simulink model "Task2_Question1"  (Simulink 8.1)
settings: Solver=FixedStepDiscrete  SolverMode=SingleTasking  StartTime=0.0  StopTime=inf  FixedStep=5e-05  RelTol=1e-3
undefined symbols (not defined in the file or in its folder): dfilt, gcbh, samplefreq, stemdo, upstartman
libraries: dspsigops x6, dsparch4 x4, dspsrcs4 x3, dspmathops x1
(part 1 of 2)
settings Model: Creator=hasan  LastModifiedBy=hasan
settings DataIOCC: SignalLoggingSaveFormat=Dataset  SaveOutput=off  SaveTime=off
settings OptimizationCC: BooleanDataType=off  ExpressionDepthLimit=128
settings DebuggingCC: MultiTaskDSMMsg=warning  FcnCallInpInsideContextMsg=EnableAllAsError  FrameProcessingCompatibilityMsg=none
settings GRTTargetCC: CombineOutputUpdateFcns=on  GRTInterface=off

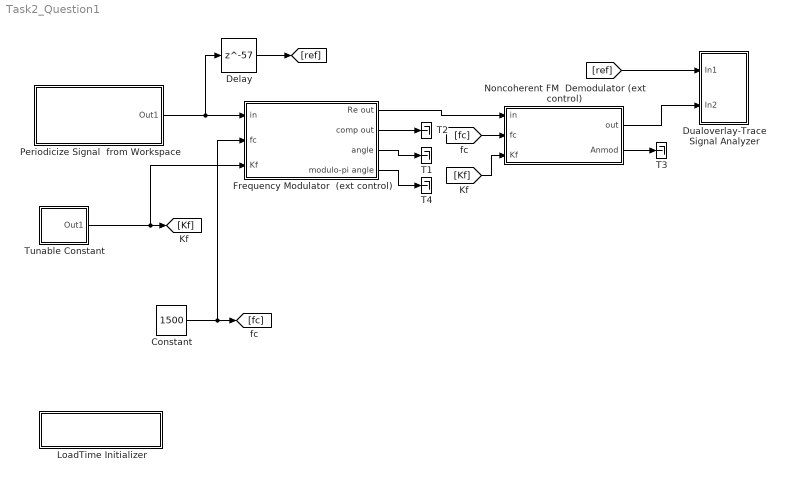
== system Task2_Question1 ==
  Constant : Constant  Value=1500
  Delay : Delay  DelayLength=57  InitialCondition=0
  Dualoverlay-Trace Signal Analyzer : Subsystem  Tag=D  Description=2-Trace Signal Analyzer (A04)  StartFcn=scopopen_April04 StartFcn  StopFcn=scopopen_April04 StopFcn  mask(2-Trace Signal Analyzer (A08)){name_plot=D, N=300, stemchoice=Continuous-plot both Inputs, V=0, nontaker=off, figpos=[0.2589 0.0583 0.6963 0.8], freqtickvec=[], strtman=off}
      mask prompts: name_plot "Name of Figure"; N "Buffer size:"; stemchoice "Plot style:"; V "Buffer overlap:"; nontaker "Override default Figure Position"; figpos "Figure Position:"; freqtickvec "Frequency-axis ticks (normally [] for default scheme)"; strtman "Startup with manual scaling"
      mask help:
      | Displays two signal vectors (depending on the choice of buffering) and their spectra. The Analyzer "name" (Name of Figure) is best assigned by clicking on the line coming into the Analyzer and labelling that line. Failing that, the dialog entry for Name of Figure is taken. If this Name collides with another Analyzer instance with the same Name, then a number is automatically added. In summary, it is permissible to give no thought to naming, unless you desire a meaningful name.
      |
      | Buffer size (typically 300) determines the number of time samples displayed and has crucial influence on stabilty of the display trace for several input sources. Both inputs (together) can either be sample-based or frame-based (when frame size matches Buffer size).
      |
      | Spectral displays can be true-zoomed in frequency (since Chirp-Z analysis is employed) via the edit boxes along the GUI bottom. By contrast, the Zoom menu item merely gives graphical zooming.
      |
      | Several controls specify the upper input port ("y" for yellow plot line) or the lower port ("w" for white plot line). Each line keeps its true vertical scaling unless temporarily overriden for VISUAL comparison purposes (see "plot scaling" menu item).
      |
      | Changes like freqtickvec and start up manual require the model to be killed and brought back up.
      | (See Help for more)
      mask init:
      | scopmsk
      settings: CopyFcn=set_param(gcb,'tag','')  DeleteFcn="scopopen_April04  DeleteFcn"  OpenFcn=scopopen_April04 OpenFcn
      mask Help:
      | Displays a signal vector (depending on the choice of buffering) and its spectrum. The Analyzer "name" (Name of Figure) is best assigned by clicking on the line coming into the Analyzer and labelling that line. Failing that, the dialog entry for Name of Figure is taken. If this Name collides with another Analyzer instance with the same Name, then a number is automatically added. In summary, it is permissible to give no thought to naming, unless you desire a meaningful name.
      | 
      | Buffer size (typically 300) determines the number of time samples displayed and has crucial influence on stabilty of the display trace for several input sources. Both inputs (together) can either be sample-based or frame-based (when frame size matches Buffer size).
      | 
      | Spectral displays can be true-zoomed in frequency (since Chirp-Z analysis is employed) via the edit boxes along the GUI bottom. By contrast, the Zoom menu item merely gives graphical zooming.
      | 
      | Several controls specify the upper input port ("y" for yellow plot line) or the lower port ("w" for white plot line). Each line keeps its true vertical scaling unless temporarily overriden for VISUAL comparison purposes (see "plot scaling" menu item).
      | 
      | Changes like freqtickvec and start up manual require the model to be killed and brought back up.
      | 
      | Dynamic amplitude scaling is automatic, but has thresholds of sensitivity (see "plot scaling" menu item) to reduce re-scale flicker . Manual re-scale (by pressing the "Full-Scale All" pushbutton is always permissible).
      | 
      | Signal (or Spectral) Averaging either uses Fading Memory from trace-to-trace (with "forgetting factor" rho unity or less) or takes each trace full-strength (over a window of N adjacent traces).
      | 
      | Copyright(c) DSP Creations Ltd. 2003-2008.
      mask TypeOptions stemchoice: Continuous-plot both Inputs | Stem-plot Input 1  [yellow]   (but 2 is continuous) | Stem-plot Input 2    [white]   (but 1 is continuous)
      mask Callback nontaker: srvscopeposition
      mask Display:
      | plot([-25 NaN 125],[0  NaN 0]);plot(0,0,100,100,[8 8 92 92 8],[92 40 40 92 92],[16 16 84],[88 48 48],[53 47 41 47 47],[34 34 34 34 21],[16 20 24 28 32 36 40 44 48 52 56 60 64 68 72 76 80],[68 74 78 80 81 80 77 73 68 64 60 58 57 57 59 63 68]);disp(name_plot);plot(0,0,100,-100,[8 8 92 92 8],-[92 40 40 92 92],[16 16 84],-[48 88 88],[24 24],-[88 58],[32 32 32],-[88 60 60],[40 40],-[88 65],[40 40],-[88 69],[48 48],-[88 80],[56 56],-[88 48],[64 64],-[88 70],[80 80 80 80],-[49 49 48 48],[53 47 47 51 47 47],-[23 23 28 28 28 34]);plot(xx,50*yy+60)
      | port_label('input',1,'y')
      | port_label('input',2,'w')
  Frequency Modulator  (ext control) : Subsystem  mask(Frequency Modulator (ext control)){thetadeg=0, sampperfr=1, twiceflag=off, conti=off, ist=off}
      mask prompts: thetadeg "Phase offset, degrees:"; sampperfr "Samples per frame"; twiceflag "Output TWICE real part (instead of Re)"; conti "Emulate continuous integration"; ist "Adopt synthetic delay-compensated time origin"
      mask help:
      | This block provides frequency modulation of a REAL signal. Both complex modulation output and real modulation are delivered.
      | The input is usually accumulated to emulate continuous-time integration. If the checkbox is on, we instead use an ABC integrator in order to more fully approximate the integration process.
      |
      | Both have had  the time origin fiddled to compensate out the group delay of the integration filter.(This is employed only if "Adopt" checkbox is ticked).
      |
      | Outputs are provided to show the instantaneous phase theta (in degrees) in exp j(2*pi*fc*t+theta(t)+ thetaoffset ), where theta emerges from our integrator  (full & modulo-pi). Note that theta seems to be on time for accumulator; must go 2 samples more for ABC integrator). That is the "comp" output.
      |
      | The real part of that is (2*pi*fc*t+theta(t)+ thetaoffset ) is delivered at the upper output port.
      | If the checkbox is ticked, then twice the real part (useful for spectral comparison) is output.
      |
      | If sample-based operation is desired then the dialog Samples per frame entry should be 1.
      |
      | The user inputs the carrier frequency through input port "fc", and the FREQUENCY SENSITIVITY (Hz/volt) through port "Kf".
      | The frequency deviation deltaf=Kf*A, when the input is a sinewave of amplitude A, as per definitions from Haykin,S.," Communication Systems",4th Edition, Wiley,2001, page 110.
      mask init:
      | sample_time_str=get_param(bdroot(gcbh),'fixedstep');
      | ts=eval(sample_time_str,'0');
      | if ts==0;
      |    samplefreq=20000;
      | else
      |    samplefreq=1/ts;
      | end;
      | a=[1 -1];
      | icvec=0;
      | b=1;
      | offs=0.5;
      | if(conti);
      |    b=[-.0099827 .0694943 .8809768  .0694943 -.0099827 ];
      |   offs=-1.5;
      | end;
      | if(~ist);offs=0;end
      | resay='Re';
      | mult=1;
      | if(twiceflag)
      | 	resay='2 Re';
      | 	mult=2;
      | end
      mask Help:
      | This block provides frequency modulation of a REAL signal. Both complex modulation output and real modulation are delivered.
      | The input is usually accumulated to emulate continuous-time integration. If the checkbox is on, we instead use an ABC integrator in order to more fully approximate the integration process.
      | 
      | Both have had  the time origin fiddled to compensate out the group delay of the integration filter.(This is employed only if "Adopt" checkbox is ticked).
      | 
      | Outputs are provided to show the instantaneous phase theta (in degrees) in exp j(2*pi*fc*t+theta(t)+ thetaoffset ), where theta emerges from our integrator  (full & modulo-pi). Note that theta seems to be on time for accumulator; must go 2 samples more for ABC integrator). That is the "comp" output.
      | 
      | The real part of that is (2*pi*fc*t+theta(t)+ thetaoffset ) is delivered at the upper output port.
      | If the checkbox is ticked, then twice the real part (useful for spectral comparison) is output.
      | 
      | If sample-based operation is desired then the dialog Samples per frame entry should be 1.
      | 
      | The user inputs the carrier frequency through input port "fc", and the FREQUENCY SENSITIVITY (Hz/volt) through port "Kf".
      | The frequency deviation deltaf=Kf*A, when the input is a sinewave of amplitude A, as per definitions from Haykin,S.," Communication Systems",4th Edition, Wiley,2001, page 110.
      | 
      | Copyright(c) DSP Creations Ltd. 2003-2013.
      mask Display:
      | disp(['Frequency\nModulator\nthetaoffset = ',num2str(thetadeg)])
      | port_label('input',1,'in')
      | port_label('input',2,'fc')
      | port_label('input',3,'Kf')
      | port_label('output',1,resay)
      | port_label('output',2,'comp')
      | port_label('output',3,'angle')
      | port_label('output',4,'mod-pi ang')
  LoadTime Initializer : Subsystem  Description="Click on block OR right-click and select \"Mask Parameters...\" for description of block."  InitFcn=eval(['load ',get_param(gcbh,'filename')])  mask(LoadTime Initializer){filename=bussgangwanderwave}
      mask prompts: filename "Specify MAT filename to load"
      mask help: Insertion of this block into a model ensures loading of the specified mat-file at load time.
      mask init:
      | linkbreakergraceful
      | eval(['load ',filename])
      mask Help:
      | Insertion of this block into a model ensures loading of the specified mat-file at load time.
      | 
      | 14_feb11
      | Copyright(c) DSP Creations Ltd. 2003-2014.
      mask Callback filename: eval(['load ',get_param(gcbh,'filename')])
      mask Display: disp(['Initialize\n '' ',filename,' '''])
  Noncoherent FM  Demodulator (ext control) : Subsystem  mask(Noncoherent FM Demodulator (ext control)){dclength=300, incomplex=off, iee=off}
      mask prompts: dclength "D.c. bias removal data block length"; incomplex "Take input as fully complex"; iee "Compensate emulation of continuous integration"
      mask help:
      | This block provides non-coherent demodulation of a real cosine frequency-modulated carrier OR frequency-modulated complex sinusoidal carrier.
      | If a fully complex input situation is known to prevail, then check  "Take input as fully complex " (which disturbs the input minimally).
      |
      | The Analyticized modulation signal is provided for viewing at the "Anmod" output port.
      |     (In case  "Take input as fully complex" is ticked, the unmodified input signal will be seen as "Anmod" ).
      |
      | The user inputs the carrier frequency through input port "fc", and the FREQUENCY SENSITIVITY (Hz/volt) through port "Kf".
      | The frequency deviation deltaf=Kf*A, when the input is a sinewave of amplitude A, as per definitions from Haykin,S.," Communication Systems",4th Edition, Wiley,2001, page 110.
      |
      | If for any reason you wish to remove all d.c. from any output, place an integer number in for "D.c. bias removal data block length". If you are satisfied with the d.c. value, instead place empty brackets for this value.
      |
      | NOTE: There is an internal 100-sample delay due to the necessary high-grade Analytic filtering. HOWEVER, if input is taken as complex there is zero delay.
      |
      | Usually the original FM signal was created by accumulation, so output is okay. But you might be working with FM where "continuous integration" had been emulated; if so, tick the last checkbox (dubious improvement).
      |
      | This demodulator requires no major bandwidth assumptions. However, the Analytic filter will give distortion if the lower bandedge of the bandpass modulation signal input is below 0.037*fs or above 0.466*fs.
      mask init:
      | linkbreakergraceful;
      | sample_time_str=get_param(bdroot(gcbh),'fixedstep');
      | ts=eval(sample_time_str,'0');
      | if ts==0;
      |    samplefreq=20000;
      | else
      |    samplefreq=1/ts;
      | end;
      | saystr=['Noncoherent FM\nDemodulator'];
      | lengthflag=0;
      | block=1;
      | if(~isempty(dclength))
      |    lengthflag=1;
      |    block=dclength;
      |    saystr=[saystr '\nd.c. remove ',num2str(dclength),'\n'];
      | end
      | bcomp=1;
      | if(iee);
      |    bint=[-.0099827 .0694943 .8809768  .0694943 -.0099827 ];
      |    bcomp=firinvleastsq(bint);
      | end;
      | insay='in';
      | if(incomplex)
      |    insay='comp in';
      | end
      mask Help:
      | This block provides non-coherent demodulation of a real cosine frequency-modulated carrier OR frequency-modulated complex sinusoidal carrier.
      | If a fully complex input situation is known to prevail, then check  "Take input as fully complex " (which disturbs the input minimally).
      | 
      | The Analyticized modulation signal is provided for viewing at the "Anmod" output port.
      |     (In case  "Take input as fully complex" is ticked, the unmodified input signal will be seen as "Anmod" ).
      | 
      | The user inputs the carrier frequency through input port "fc", and the FREQUENCY SENSITIVITY (Hz/volt) through port "Kf".
      | The frequency deviation deltaf=Kf*A, when the input is a sinewave of amplitude A, as per definitions from Haykin,S.," Communication Systems",4th Edition, Wiley,2001, page 110.
      | 
      | If for any reason you wish to remove all d.c. from any output, place an integer number in for "D.c. bias removal data block length". If you are satisfied with the d.c. value, instead place empty brackets for this value.
      | 
      | NOTE: There is an internal 100-sample delay due to the necessary high-grade Analytic filtering. HOWEVER, if input is taken as complex there is zero delay.
      | 
      | Usually the original FM signal was created by accumulation, so output is okay. But you might be working with FM where "continuous integration" had been emulated; if so, tick the last checkbox (dubious improvement).
      | 
      | This demodulator requires no major bandwidth assumptions. However, the Analytic filter will give distortion if the lower bandedge of the bandpass modulation signal input is below 0.037*fs or above 0.466*fs.
      | 
      | 14_May5
      | Copyright(c) DSP Creations Ltd. 2003-2014.
      mask Display:
      | disp(saystr)
      | port_label('input',1,insay)
      | port_label('input',2,'fc')
      | port_label('input',3,'Kf')
      | port_label('output',1,'out')
      | port_label('output',2,'Anmod')
  Periodicize Signal  from Workspace : Subsystem  mask(Arbitrary Periodic Signal Generator){signal_name_str=bussgangwanderwave, A=1, Ntry=[], dwellsamp=1, fill0=off}
      mask prompts: signal_name_str "Signal name (in workspace)"; A "Amplification, A"; Ntry "Period, N (=[ ] if same as length of signal)"; dwellsamp "Dwell interval (in samples) before stepping to next sample of signal"; fill0 "Fill interval between signal samples with zeros (instead of holding)"
      mask help:
      | This takes a vector signal in the workspace as the base period for a periodic signal. Note that a short period can time-alias the base period. At present, no special icon indication comes if the signal is complex.
      |
      | This signal generator is analogous to a Refresh DAC; it loads in (from the Workspace or from its dialog box) a (real or complex) signal vector and then repeatedly clocks it out. We have really a causal periodic buildup. Normally you let the vector "Signal name" dictate the period (to be length of signal_name) by leaving "Period" empty, but this can be set longer or (if shorter) to time-alias. Note that a vector of numbers can be used in place of a vector name in the dialog box.
      |
      | Dwell interval (usually 1 when stepping right through signal samples), dwellsamp, can be set to an integer value. This then holds the signal value constant for dwellsamp clock times before moving on to take the next sample explicitly set out in  the vector signal name.
      | Thus, the true period taken to cycle through the signal is  Period*dwellsamp.
      |
      | If the checkbox is ticked the dwellsample interval between specified signal samples is filled with zeros; otherwise values are held for whole interval.
      mask init:
      | maskmaster('passkey_integerize','Ntry',Ntry);
      | sample_time_str=get_param(bdroot(gcbh),'fixedstep');
      | ts=eval(sample_time_str,'0');
      | if ts==0;
      |    samplefreq=20000;
      | else
      |    samplefreq=1/ts;
      | end;
      | signal_name=evalin('base',signal_name_str,'[1:4]');
      | Ns=length(signal_name);
      | if(isempty(Ntry))
      |    N=Ns;
      | else
      |    N=Ntry;
      | end
      | if(Ns<=N);
      |     x=[signal_name  zeros(1,N-Ns)];
      | else;
      |     innn=[signal_name zeros(1,Ns+2*N)];
      |     opt=filter(1,[1 zeros(1,N-1) -1],innn);
      |     x=opt(length(signal_name)+1:Ns+2*N);
      | end
      | iflag=0;
      | if(any(imag(x)))
      |   iflag=1;
      | end
      | if(isreal(x))
      |   d2=['total cycle= ' num2str(N*dwellsamp)];
      | else	
      |   d2=['total cycle= ' num2str(N*dwellsamp),'   (Re seen)'];
      | end
      | dwellsamp=floor(abs(dwellsamp));
      | gg=real(x);
      | Lg=length(gg);
      | rr=repmat(gg,dwellsamp,1);
      | zerodo=0;
      | if(strcmp(fill0,'on'));
      | 	zerodo=1;	
      |    rr=[gg; zeros(dwellsamp-1,Lg)];
      | end 
      | gg=reshape(rr,1,dwellsamp*Lg);
      | if(length(gg)>2000)
      |    dec=ceil(length(gg)/2000);
      |    gg=gg(1:dec:end);
      | end	
      | mm=max(gg);
      | mi=min(gg);
      | Ngg=length(gg);
      mask Help:
      | This takes a vector signal in the workspace as the base period for a periodic signal. Note that a short period can time-alias the base period. At present, no special icon indication comes if the signal is complex.
      | 
      | This signal generator is analogous to a Refresh DAC; it loads in (from the Workspace or from its dialog box) a (real or complex) signal vector and then repeatedly clocks it out. We have really a causal periodic buildup. Normally you let the vector "Signal name" dictate the period (to be length of signal_name) by leaving "Period" empty, but this can be set longer or (if shorter) to time-alias. Note that a vector of numbers can be used in place of a vector name in the dialog box.
      | 
      | Dwell interval (usually 1 when stepping right through signal samples), dwellsamp, can be set to an integer value. This then holds the signal value constant for dwellsamp clock times before moving on to take the next sample explicitly set out in  the vector signal name.
      | Thus, the true period taken to cycle through the signal is  Period*dwellsamp.
      | 
      | If the checkbox is ticked the dwellsample interval between specified signal samples is filled with zeros; otherwise values are held for whole interval.
      | 
      | 14_Feb12
      | Copyright(c) DSP Creations Ltd. 2003-2014.
      mask Display:
      | plot(.02+.96*[0:Ngg-1]/(Ngg-1),.28+.6*(gg-mi)/(mm-mi))
      | text(.02,.9,[signal_name_str,' periodicized'])
      | text(.02,.255,['period= ' num2str(N) ' samples'])
      | text(.02,.085,d2)
  T{1..4} (4 alike) : Terminator
  Tunable Constant : Subsystem  LoadFcn=slideg Load  mask(Tunable Constant){low=0, gain=3397, high=3397}
      mask help: This signal generator gives out a constant value which is slider-adjustable.
      mask init:
      | %set_param(gcb,'linkstatus','none');
      | if(~strcmp(get_param(gcb,'linkstatus'),'none'))
      |    set_param(gcb,'linkstatus','none');	
      | end
      | sample_freq=maskmaster('Sinusoid Generator',1);
      settings: CopyFcn=slideg Copy  DeleteFcn=slideg DeleteBlock  NameChangeFcn=slideg NameChange  OpenFcn=slideg Open  CloseFcn=slideg Close  ParentCloseFcn=slideg ParentClose
      mask Help:
      | This signal generator gives out a constant value which is slider-adjustable.
      | 
      | Copyright(c) DSP Creations Ltd. 2003-2013.
      mask Display: disp(gain)
  wires:
  Frequency Modulator  (ext control)/2(comp out) -> T2/1
  Frequency Modulator  (ext control)/3(angle) -> T1/1
  Frequency Modulator  (ext control)/4(modulo-pi angle) -> T4/1
  Noncoherent FM  Demodulator (ext control)/2(Anmod) -> T3/1
  Periodicize Signal  from Workspace/1(Out1) -> Delay/1, Frequency Modulator  (ext control)/1(in)
  Frequency Modulator  (ext control)/1(Re out) -> Noncoherent FM  Demodulator (ext control)/1(in)
  Constant/1 -> [fc], Frequency Modulator  (ext control)/2(fc)
  Delay/1 -> [ref]
  [ref] -> Dualoverlay-Trace Signal Analyzer/1(In1)
  Noncoherent FM  Demodulator (ext control)/1(out) -> Dualoverlay-Trace Signal Analyzer/2(In2)
  Tunable Constant/1(Out1) -> [Kf], Frequency Modulator  (ext control)/3(Kf)
  [fc] -> Noncoherent FM  Demodulator (ext control)/2(fc)
  [Kf] -> Noncoherent FM  Demodulator (ext control)/3(Kf)

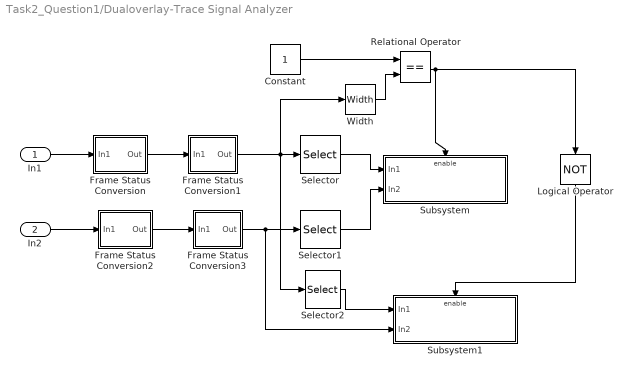
== system Task2_Question1/Dualoverlay-Trace Signal Analyzer ==
  In1 : Inport
  In2 : Inport  Port=2
  Constant : Constant
  Frame Status Conversion : Subsystem  mask(Frame Status Conversion){growRefPort=off, outframe=Frame-based}
      mask prompts: growRefPort "Inherit output frame status from Ref input port"; outframe "Output signal:"
      mask help: Specify the frame status of the output signal.
      mask init:
      | [p, str] = dspblkfrmconv('init');
      mask Help: web(dspbhelp);
      mask Callback growRefPort: dspblkfrmconv
      mask TypeOptions outframe: Frame-based | Sample-based
      mask Display:
      | port_label(p.in1,   p.i1,  p.i1s);
      | port_label(p.in2,   p.i2,  p.i2s);
      | port_label(p.out, p.o1, p.o1s);
      | disp(str)
  Frame Status Conversion1 : Subsystem  mask(Frame Status Conversion){growRefPort=off, outframe=Sample-based}
      mask prompts: growRefPort "Inherit output frame status from Ref input port"; outframe "Output signal:"
      mask help: Specify the frame status of the output signal.
      mask init:
      | [p, str] = dspblkfrmconv('init');
      mask Help: web(dspbhelp);
      mask Callback growRefPort: dspblkfrmconv
      mask TypeOptions outframe: Frame-based | Sample-based
      mask Display:
      | port_label(p.in1,   p.i1,  p.i1s);
      | port_label(p.in2,   p.i2,  p.i2s);
      | port_label(p.out, p.o1, p.o1s);
      | disp(str)
  Frame Status Conversion2 : Subsystem  mask(Frame Status Conversion){growRefPort=off, outframe=Frame-based}
      mask prompts: growRefPort "Inherit output frame status from Ref input port"; outframe "Output signal:"
      mask help: Specify the frame status of the output signal.
      mask init:
      | [p, str] = dspblkfrmconv('init');
      mask Help: web(dspbhelp);
      mask Callback growRefPort: dspblkfrmconv
      mask TypeOptions outframe: Frame-based | Sample-based
      mask Display:
      | port_label(p.in1,   p.i1,  p.i1s);
      | port_label(p.in2,   p.i2,  p.i2s);
      | port_label(p.out, p.o1, p.o1s);
      | disp(str)
  Frame Status Conversion3 : Subsystem  mask(Frame Status Conversion){growRefPort=off, outframe=Sample-based}
      mask prompts: growRefPort "Inherit output frame status from Ref input port"; outframe "Output signal:"
      mask help: Specify the frame status of the output signal.
      mask init:
      | [p, str] = dspblkfrmconv('init');
      mask Help: web(dspbhelp);
      mask Callback growRefPort: dspblkfrmconv
      mask TypeOptions outframe: Frame-based | Sample-based
      mask Display:
      | port_label(p.in1,   p.i1,  p.i1s);
      | port_label(p.in2,   p.i2,  p.i2s);
      | port_label(p.out, p.o1, p.o1s);
      | disp(str)
  Logical Operator : Logic  Operator=NOT
  Relational Operator : RelationalOperator  Operator===  InputSameDT=on
  Selector : Selector  NumberOfDimensions=2  InputPortWidth=3  IndexOptions=Index vector (dialog),Index vector (dialog)  Indices=1,1  OutputSizes=1
  Selector1 : Selector  NumberOfDimensions=2  InputPortWidth=3  IndexOptions=Index vector (dialog),Index vector (dialog)  Indices=1,1  OutputSizes=1
  Selector2 : Selector  NumberOfDimensions=2  InputPortWidth=3  IndexOptions=Select all,Index vector (dialog)  Indices=-1,1  OutputSizes=1
  Subsystem : Subsystem  TreatAsAtomicUnit=on
  Subsystem1 : Subsystem  TreatAsAtomicUnit=on
  Width : Width
  wires:
  Selector1/1 -> Subsystem/2(In2)
  Selector/1 -> Subsystem/1(In1)
  Selector2/1 -> Subsystem1/1(In1)
  Logical Operator/1 -> Subsystem1/Enable
  Relational Operator/1 -> Logical Operator/1, Subsystem/Enable
  Width/1 -> Relational Operator/2
  Constant/1 -> Relational Operator/1
  Frame Status Conversion3/1(Out) -> Subsystem1/2(In2), Selector1/1
  In2/1 -> Frame Status Conversion2/1(In1)
  Frame Status Conversion2/1(Out) -> Frame Status Conversion3/1(In1)
  Frame Status Conversion1/1(Out) -> Selector2/1, Selector/1, Width/1
  In1/1 -> Frame Status Conversion/1(In1)
  Frame Status Conversion/1(Out) -> Frame Status Conversion1/1(In1)

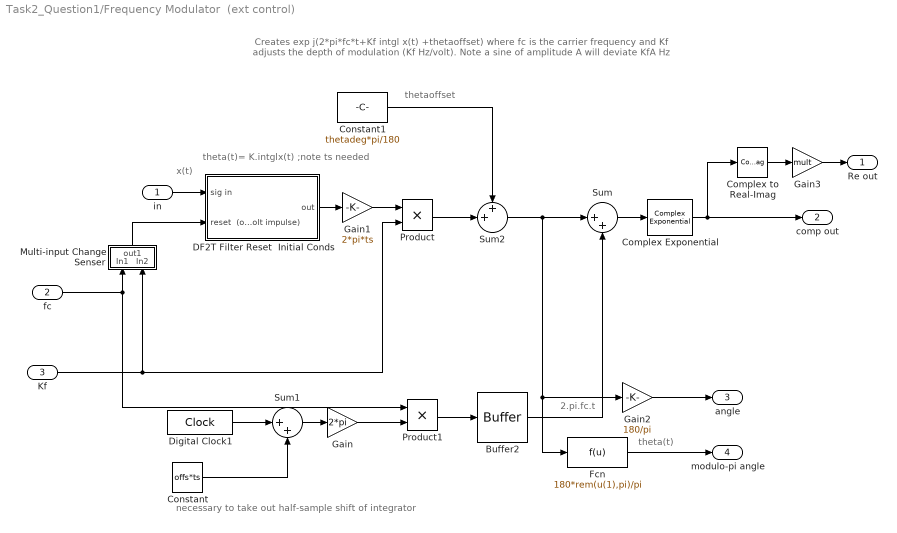
== system Task2_Question1/Frequency Modulator  (ext control) ==
  note: thetaoffset
  note: x(t)
  note: Creates exp j(2*pi*fc*t+Kf intgl x(t) +thetaoffset) where fc is  the carrier frequency
      |  and Kf adjusts the depth of modulation (Kf Hz/volt).
      |  Note a sine of amplitude A will deviate KfA Hz
  note: 2.pi.fc.t
  note: theta(t)=
      | K.intglx(t) ;note ts needed
  note: necessary to take out
      |  half-sample shift of integrator
  note: theta(t)
  in : Inport
  fc : Inport  Port=2
  Kf : Inport  Port=3
  Buffer2 : Buffer  N=sampperfr
  Complex Exponential : dspmathops/Complex Exponential
  Complex to Real-Imag : ComplexToRealImag  Output=Real
  Constant : Constant  Value=offs*ts
  Constant1 : Constant  Value=thetadeg*pi/180
  DF2T Filter Reset  Initial Conds : Subsystem  mask(Direct Form 2 Transpose Filter Reset Initial Conds){b=b, a=a, Xicvec=0, Yicvec=0}
      mask prompts: b "Numerator coefficient vector, b"; a "Denominator coefficient vector, a"; Xicvec "Vector of  INPUT x initial conditions, Xicvec:"; Yicvec "Vector of  OUTPUT y initial conditions, Yicvec:"
      mask help:
      | This block has resettable initial conditions, making it possible to exhibit stationary repetitive displays of the effects of ic's, perhaps even as coefficients are tuned.
      |
      | The b and a filter  coefficients are input as vector parameters.
      | The initial condition vectors  are fed in in this form:
      |    Xicvec = [ x[-1] x[-2] x[-3] ... x[-nb] ... ]   (inputs)
      |    Yicvec = [ y[-1] y[-2] y[-3] ... y[-na] ... ]    (outputs)
      |
      | (These are packaged for DF2T as a chain of delayor ic's internal to the block, using MATLAB's filtic command).
      |
      | The output of the filter is delayed by one bulk sample  since, internal to this block, the reset has to initiate immediately (before data flow).
      | (That is, the first sample out of the filter is actually y(-1), so there is a pervasive delay of the time scale by one sample.
      |
      | Resetting is achieved by a unit-amplitude impulse.
      mask init:
      | icvec=filtic(b,a,Yicvec,Xicvec);
      | sample_time_str=get_param(bdroot(gcbh),'fixedstep');
      | ts=eval(sample_time_str,'0');
      | if ts==0;
      |    samplefreq=20000;
      | else
      |    samplefreq=1/ts;
      | end;
      mask Help:
      | This block has resettable initial conditions, making it possible to exhibit stationary repetitive displays of the effects of ic's, perhaps even as coefficients are tuned.
      | 
      | The b and a filter  coefficients are input as vector parameters.
      | The initial condition vectors  are fed in in this form:
      |    Xicvec = [ x[-1] x[-2] x[-3] ... x[-nb] ... ]   (inputs)
      |    Yicvec = [ y[-1] y[-2] y[-3] ... y[-na] ... ]    (outputs)
      | 
      | (These are packaged for DF2T as a chain of delayor ic's internal to the block, using MATLAB's filtic command).
      | 
      | The output of the filter is delayed by one bulk sample  since, internal to this block, the reset has to initiate immediately (before data flow).
      | (That is, the first sample out of the filter is actually y(-1), so there is a pervasive delay of the time scale by one sample.
      | 
      | Resetting is achieved by a unit-amplitude impulse.
      | 
      | Copyright(c) DSP Creations Ltd. 2003-2006.
      mask Display:
      | disp('Direct Form 2T\nReset Initial\nCond Filter')
      | port_label('input',1,'in')
      | port_label('input',2,'reset')
  Digital Clock1 : DigitalClock  SampleTime=ts
  Fcn : Fcn  Expr=180*rem(u(1),pi)/pi
  Gain : Gain  Gain=2*pi  SaturateOnIntegerOverflow=on  OutDataTypeStr=Inherit: Same as input  ParamDataTypeStr=Inherit: Same as input
  Gain1 : Gain  Gain=2*pi*ts  SaturateOnIntegerOverflow=on  OutDataTypeStr=Inherit: Same as input  ParamDataTypeStr=Inherit: Same as input
  Gain2 : Gain  Gain=180/pi  SaturateOnIntegerOverflow=on  OutDataTypeStr=Inherit: Same as input  ParamDataTypeStr=Inherit: Same as input
  Gain3 : Gain  Gain=mult  SaturateOnIntegerOverflow=on  OutDataTypeStr=Inherit: Same as input  ParamDataTypeStr=Inherit: Same as input
  Multi-input Change Senser : Subsystem  Description=Multi-Input Change Senser  mask(Multi-input Change Senser){vector=[1 2]}
      mask prompts: vector "Channel Values Vector"
      mask help:
      | This block detects any change on any of its input ports (including at startup) and issues a unit-voltage impulse.
      |
      | The syntax for the Channel Values Vector is, e.g.: [1 2 3 4] or [5 8]:
      |
      | WARNING: Any block housing this block should itself initialize with set_param(gcb,'linkstatus','none');
      mask init:
      | set_param(gcb,'linkstatus','none');
      mask Help:
      | This block detects any change on any of its input ports (including at startup) and issues a unit-voltage impulse.
      | 
      | The syntax for the Channel Values Vector is, e.g.: [1 2 3 4] or [5 8]:
      | 
      | WARNING: Any block housing this block should itself initialize with set_param(gcb,'linkstatus','none');
      | 
      | Copyright(c) DSP Creations Ltd. 2003-2010.
      mask Callback vector: udscope3d_forsenser
      mask Display: port_label('input',1,'1'),port_label('input',2,'2'),
  Product : Product  SaturateOnIntegerOverflow=on  OutDataTypeStr=Inherit: Same as first input
  Product1 : Product  SaturateOnIntegerOverflow=on  OutDataTypeStr=Inherit: Same as first input
  Sum : Sum  Inputs=|++  SaturateOnIntegerOverflow=on  InputSameDT=on  OutDataTypeStr=Inherit: Same as first input
  Sum1 : Sum  Inputs=|++  SaturateOnIntegerOverflow=on  InputSameDT=on  OutDataTypeStr=Inherit: Same as first input
  Sum2 : Sum  Inputs=++|  SaturateOnIntegerOverflow=on  InputSameDT=on  OutDataTypeStr=Inherit: Same as first input
  Re out : Outport  InitialOutput=0
  comp out : Outport  Port=2  InitialOutput=0
  angle : Outport  Port=3  InitialOutput=0
  modulo-pi angle : Outport  Port=4  InitialOutput=0
  wires:
  fc/1 -> Product1/1, Multi-input Change Senser/1(In1)
  Product1/1 -> Buffer2/1
  Gain/1 -> Product1/2
  Kf/1 -> Multi-input Change Senser/2(In2), Product/2
  Product/1 -> Sum2/2
  Gain1/1 -> Product/1
  Multi-input Change Senser/1(out1) -> DF2T Filter Reset  Initial Conds/2(reset  (one-volt impulse))
  Constant1/1 -> Sum2/1
  Sum2/1 -> Gain2/1, Fcn/1, Sum/1
  Gain3/1 -> Re out/1
  Complex to Real-Imag/1 -> Gain3/1
  Complex Exponential/1 -> Complex to Real-Imag/1, comp out/1
  in/1 -> DF2T Filter Reset  Initial Conds/1(sig in)
  DF2T Filter Reset  Initial Conds/1(out) -> Gain1/1
  Sum/1 -> Complex Exponential/1
  Fcn/1 -> modulo-pi angle/1
  Gain2/1 -> angle/1
  Digital Clock1/1 -> Sum1/1
  Sum1/1 -> Gain/1
  Constant/1 -> Sum1/2
  Buffer2/1 -> Sum/2

== system Task2_Question1/LoadTime Initializer ==

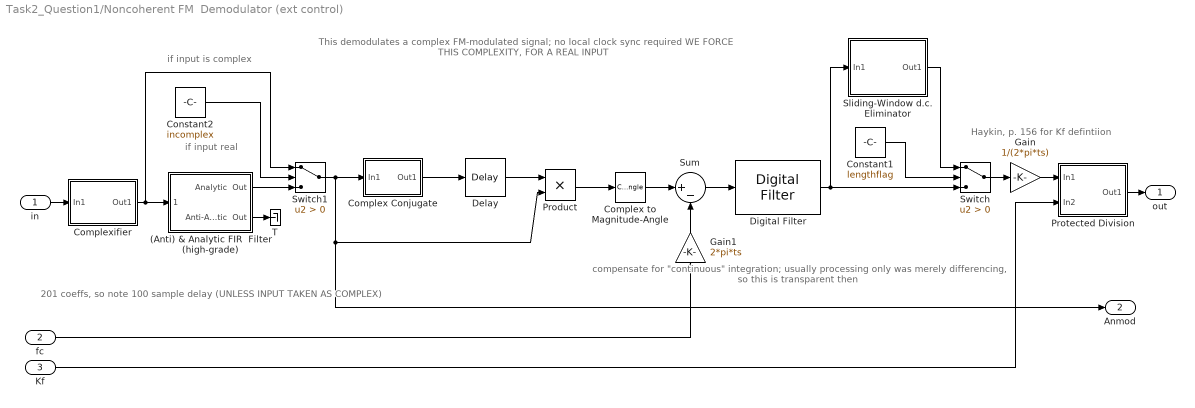
== system Task2_Question1/Noncoherent FM  Demodulator (ext control) ==
  note: This demodulates a complex FM-modulated signal; no local clock sync required
      | WE FORCE THIS COMPLEXITY, FOR A REAL INPUT
  note: compensate for "continuous" integration;
      | usually processing only was
      |  merely differencing, so this is
      | transparent then
  note: Haykin, p. 156
      |  for Kf defintiion
  note: 201 coeffs, so note
      |  100 sample delay
      | (UNLESS INPUT
      |  TAKEN AS COMPLEX)
  note: if input is complex
  note: if input real
  in : Inport
  fc : Inport  Port=2
  Kf : Inport  Port=3
  (Anti) & Analytic FIR  Filter (high-grade) : Subsystem  Description=|  mask((Anti) and Analytic FIR Filter (high-grade)){icvec=0, opcoeffs=off}
      | This block filters just like MATLAB's filter command.The b coefficient vector is either typed in-place numerically or is the name of some vector in the Workspace.
      |                                                                                                                                                                   
      | Initial conditions are always zero.                                                                                                                               
      |                                                                                                                                                                   
      | A checkbox allows normalization of the impulse response to unit energy. A second checkbox allows creation of a port for output of the b coefficient vector.       
      |                                                                                                                                                                   
      | Copyright(c) DSP Creations Ltd. 2003-2004.
      mask prompts: icvec "Vector of  INPUT x initial conditions, Xicvec:"; opcoeffs "Output Filter Coefficients"
      mask help:
      | This block provides high-grade Analytic filtering from the upper output port. That is, for negative frequencies the gain is zero, while it is 2 for positive frequencies.
      | This a fixed design, with 201 coefficients; it has linear phase and a delay of 100 samples.
      |
      | Error is less than 0.000003 from frequency of 0.037*fs to 0.466*fs , and about symmetrically.
      | Thus, if you can live with the bandlimitedness, the quality is excellent.
      |
      | The initial condition vectors  are fed in in this form:
      |    Xicvec = [ x[-1] x[-2] x[-3] ... x[-nb] ... ]   (inputs)
      |
      | A checkbox allows creation of a port for output of the b coefficient vector.
      mask init:
      | b=analyticFIRhighgrade;
      | gg=gain(b,1);
      | if(length(gg)>2000)
      |    dec=ceil(length(gg)/2000);
      |    gg=gg(1:dec:end);
      | end	
      | mm=max(gg);
      mask Help:
      | This block provides high-grade Analytic filtering. That is, for negative frequencies the gain is zero, while it is 2 for positive frequencies.
      | This a fixed design, with 201 coefficients; it has linear phase and a delay of 100 samples.
      | 
      | Error is less than 0.000003 from frequency of 0.037*fs to 0.466*fs , and about symmetrically.
      | Thus, if you can live with the bandlimitedness, the quality is excellent.
      | 
      | The initial condition vectors  are fed in in this form:
      |    Xicvec = [ x[-1] x[-2] x[-3] ... x[-nb] ... ]   (inputs)
      | 
      | A checkbox allows creation of a port for output of the b coefficient vector.
      | 
      | Copyright(c) DSP Creations Ltd. 2003-2007.
      mask Callback opcoeffs: constructoutputs(gcb,1)
      mask Display:
      | color('blue');
      | plot([1.1*mm nan gg nan -0.1])
      | color('black');
      | text(0,-.2*mm,[' Analytic, N=201'])
      | text(0,-.4*mm,[' '])
  Complex Conjugate : Subsystem  mask(Complex Conjugate){}
      mask help: This block forms the complex conjugate of its input.
      mask Help:
      | This block forms the complex conjugate of its input.
      | 
      | Copyright(c) DSP Creations Ltd. 2003-2004.
      mask Display: disp('*\nConjugate' )
  Complex to Magnitude-Angle : ComplexToMagnitudeAngle  Output=Angle
  Complexifier : Subsystem  mask(Phoney Complexifier){}
      mask help: This utility block makes its input complex even if real. It is sometimes useful for interfacing simultaneous input with mixed real and complex types.
      mask Help:
      | This utility block makes its input  complex even if real. It is sometimes useful for interfacing simultaneous input with mixed real and complex types.
      | 
      | Copyright(c) DSP Creations Ltd. 2003-2004.
      mask Display: disp('Phoney\nComplexifier')
  Constant1 : Constant  Value=lengthflag
  Constant2 : Constant  Value=incomplex
  Delay : dspsigops/Delay  InputProcessing=Inherited (this choice will be removed - see release notes)  dly_unit=Samples  delay=1  ic_detail=off  dif_ic_for_ch=off  dif_ic_for_dly=off  ic=0  reset_popup=None
  Digital Filter : dsparch4/Digital Filter  TypePopup=FIR (all zeros)  IIRFiltStruct=Direct form II transposed  AllPoleFiltStruct=Direct form  FIRFiltStruct=Direct form  CoeffSource=Specify via dialog  NumCoeffs=bcomp  DenCoeffs=bcomp  BiQuadCoeffs=[1 0.3 0.4 1 0.1 0.2]  LatticeCoeffs=[0.2 0.4]  denIgnore=on  FiltPerSampPopup=One filter per frame  IC=0  ICnum=0  ICden=0  roundingMode=Floor  overflowMode=off  ScaleValues=1  scaleValueFracLength=14  stageInFracLength=15  stageOutFracLength=15  FilterSource=Specify via dialog  dfiltObjectName=dfilt.dffir([1 2 1])  InputProcessing=Inherited (this choice will be removed - see release notes)
  Gain : Gain  Gain=1/(2*pi*ts)  SaturateOnIntegerOverflow=on  OutDataTypeStr=Inherit: Same as input  ParamDataTypeStr=Inherit: Same as input
  Gain1 : Gain  Gain=2*pi*ts  SaturateOnIntegerOverflow=on  OutDataTypeStr=Inherit: Same as input  ParamDataTypeStr=Inherit: Same as input
  Product : Product  SaturateOnIntegerOverflow=on  InputSameDT=on  OutDataTypeStr=Inherit: Same as first input
  Protected Division : Subsystem  mask(Safe Divider){}
      mask help: This utility block protects against division by zero. The output holds at its last value whenever input "denom" takes on value zero. On the initial clock instant the output is made zero. Otherwise the output is num/denom.
      mask init:
      | linkbreakergraceful;
      mask Help:
      | This utility block protects against division by zero. The output holds at its last value whenever input "denom" takes on value zero. On the initial clock instant the output is made zero. Otherwise the output is num/denom.
      | 
      | 14_March5
      | Copyright(c) DSP Creations Ltd. 2003-2014.
      mask Display:
      | disp('\nSafe Divider\n')
      | port_label('input',1,'num')
      | port_label('input',2,'denom')
  Sliding-Window d.c. Eliminator : Subsystem  mask(Sliding Block D.C. Eliminator){N=block}
      mask prompts: N "Data block length, N"
      mask help:
      | This block removes the d.c. content from a block of data N units long. The removal is done sample-by-sample, on a sliding-window basis (with N the window length).
      |
      | The output is the current sample minus the average of all N values preceeding (and including) this sample.
      mask init:
      | sample_time_str=get_param(bdroot(gcbh),'fixedstep');
      | ts=eval(sample_time_str,'0');
      | if ts==0;
      |    samplefreq=20000;
      | else
      |    samplefreq=1/ts;
      | end;
      mask Help:
      | This block removes the d.c. content from a block of data N units long. The removal is done sample-by-sample, on a sliding-window basis (with N the window length).
      | 
      | The output is the current sample minus the average of all N values preceeding (and including) this sample.
      | 
      | Copyright(c) DSP Creations Ltd. 2003-2012.
      mask Display: disp(['N= ',num2str(N),' size\nBlock d.c.\nEliminator'])
  Sum : Sum  Inputs=|+-  SaturateOnIntegerOverflow=on  InputSameDT=on  OutDataTypeStr=Inherit: Same as first input
  Switch : Switch  Criteria=u2 > Threshold  SaturateOnIntegerOverflow=on
  Switch1 : Switch  Criteria=u2 > Threshold  SaturateOnIntegerOverflow=on
  T : Terminator
  out : Outport
  Anmod : Outport  Port=2
  wires:
  fc/1 -> Gain1/1
  Gain1/1 -> Sum/2
  Complex to Magnitude-Angle/1 -> Sum/1
  Kf/1 -> Protected Division/2(In2)
  Gain/1 -> Protected Division/1(In1)
  Protected Division/1(Out1) -> out/1
  Complexifier/1(Out1) -> Switch1/1, (Anti) & Analytic FIR  Filter (high-grade)/1(" ")
  Sliding-Window d.c. Eliminator/1(Out1) -> Switch/1
  Constant1/1 -> Switch/2
  Switch/1 -> Gain/1
  Product/1 -> Complex to Magnitude-Angle/1
  Sum/1 -> Digital Filter/1
  Digital Filter/1 -> Sliding-Window d.c. Eliminator/1(In1), Switch/3
  Delay/1 -> Product/1
  Complex Conjugate/1(Out1) -> Delay/1
  in/1 -> Complexifier/1(In1)
  Switch1/1 -> Anmod/1, Product/2, Complex Conjugate/1(In1)
  (Anti) & Analytic FIR  Filter (high-grade)/1(Analytic  Out) -> Switch1/3
  Constant2/1 -> Switch1/2
  (Anti) & Analytic FIR  Filter (high-grade)/2(Anti-Analytic  Out) -> T/1

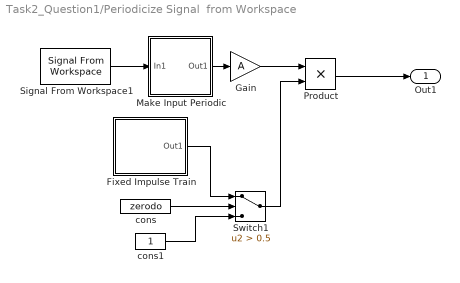
== system Task2_Question1/Periodicize Signal  from Workspace ==
  Fixed Impulse Train : Subsystem  mask(Fixed Impulse Train){N=dwellsamp}
      mask prompts: N "Repetition Period, N:"
      mask help:
      | A periodic train of unit-amplitude impulses is provided.
      |
      | This signal generator gives a unit-amplitude impulse every N samples. Intervening samples are zero-valued.
      mask init:
      | if(isempty(N))
      |     errordlg('ERROR: this value must be set to a positive integer',gcb,'modal')
      | else
      |    maskmaster('passkey_integerize','N',N)
      | end
      | sample_time_str=get_param(bdroot(gcbh),'fixedstep');
      | ts=eval(sample_time_str,'0');
      | if ts==0;
      |    samplefreq=20000;
      | else
      |    samplefreq=1/ts;
      | end;
      mask Help:
      | A periodic train of unit-amplitude impulses is provided.
      | 
      | This signal generator gives a unit-amplitude impulse every N samples. Intervening samples are zero-valued.
      | 
      | Copyright(c) DSP Creations Ltd. 2003-2004
      mask Display: disp(['Fixed Impulse\nTrain,\n Period:\n N= ',num2str(N)])
  Gain : Gain  Gain=A  SaturateOnIntegerOverflow=on  OutDataTypeStr=Inherit: Same as input  ParamDataTypeStr=Inherit: Same as input
  Make Input Periodic : Subsystem  mask(Periodicizer){N=N}
      mask prompts: N "Period  (in samples)"
      mask help: This block takes any input and (causally) constructs a periodic signal using that. Note that a short period can time-alias the base period.
      mask init:
      | if(isempty(N))
      |     errordlg('ERROR: this value must be set to a positive integer',gcb,'modal')
      | else
      |    maskmaster('passkey_integerize','N',N)
      | end
      mask Help: This auxiliary device produces a (causal) periodic buildup. Normally you let the incoming signal vector  dictate the period (by taking care to set "Period" to be the length of that vector). (See also "Periodicize Signal from Workspace" block).
      mask Display: disp(['Periodicizer\nperiod= ',num2str(N)])
  Product : Product  SaturateOnIntegerOverflow=on  OutDataTypeStr=Inherit: Same as first input
  Signal From Workspace1 : dspsrcs4/Signal From Workspace  X=signal_name  Ts=dwellsamp/samplefreq  nsamps=1  OutputAfterFinalValue=Setting to zero  ignoreOrWarnInputAndFrameLengths=off
  Switch1 : Switch  Criteria=u2 > Threshold  Threshold=0.5  SaturateOnIntegerOverflow=on
  cons : Constant  Value=zerodo
  cons1 : Constant
  Out1 : Outport  SampleTime=1/samplefreq  InitialOutput=0
  wires:
  cons1/1 -> Switch1/3
  Switch1/1 -> Product/2
  Fixed Impulse Train/1(Out1) -> Switch1/1
  Product/1 -> Out1/1
  Gain/1 -> Product/1
  cons/1 -> Switch1/2
  Make Input Periodic/1(Out1) -> Gain/1
  Signal From Workspace1/1 -> Make Input Periodic/1(In1)

== system Task2_Question1/Tunable Constant ==
  Constant : Constant  Value=gain
  Out1 : Outport
  wires:
  Constant/1 -> Out1/1

== system Task2_Question1/Dualoverlay-Trace Signal Analyzer/Frame Status Conversion ==
  In1 : Inport
  Frame Status : FrameConversion
  Out : Outport
  wires:
  Frame Status/1 -> Out/1
  In1/1 -> Frame Status/1

== system Task2_Question1/Dualoverlay-Trace Signal Analyzer/Frame Status Conversion1 ==
  In1 : Inport
  Frame Status : FrameConversion  OutFrame=Sample-based
  Out : Outport
  wires:
  Frame Status/1 -> Out/1
  In1/1 -> Frame Status/1

== system Task2_Question1/Dualoverlay-Trace Signal Analyzer/Frame Status Conversion2 ==
  In1 : Inport
  Frame Status : FrameConversion
  Out : Outport
  wires:
  Frame Status/1 -> Out/1
  In1/1 -> Frame Status/1

== system Task2_Question1/Dualoverlay-Trace Signal Analyzer/Frame Status Conversion3 ==
  In1 : Inport
  Frame Status : FrameConversion  OutFrame=Sample-based
  Out : Outport
  wires:
  Frame Status/1 -> Out/1
  In1/1 -> Frame Status/1

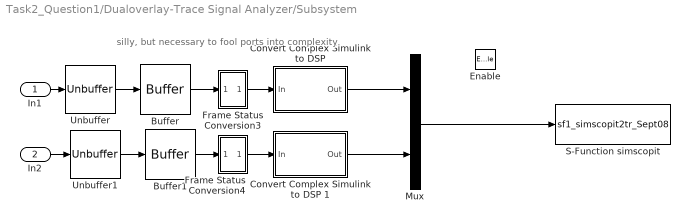
== system Task2_Question1/Dualoverlay-Trace Signal Analyzer/Subsystem ==
  note: silly, but necessary to fool ports
      | into complexity
  In1 : Inport
  In2 : Inport  Port=2
  Enable : EnablePort
  Buffer : Buffer  N=N  V=V  ic=ic
  Buffer1 : Buffer  N=N  V=V  ic=ic
  "Convert Complex Simulink to DSP " : Subsystem  mask(Convert Complex Simulink to DSP){}
      mask help: Convert new Simulink complex data type to old DSP Blockset (prior to V3.0) complex data format.
      mask init:
      | [x,y]=cplxico2(1,[]);
      mask Help: web(dspbhelp);
      mask Display:
      | plot(x,y);
      | text(10,50,'Convert\nComplex','horiz','left');
  Convert Complex Simulink to DSP 1 : Subsystem  mask(Convert Complex Simulink to DSP){}
      mask help: Convert new Simulink complex data type to old DSP Blockset (prior to V3.0) complex data format.
      mask init:
      | [x,y]=cplxico2(1,[]);
      mask Help: web(dspbhelp);
      mask Display:
      | plot(x,y);
      | text(10,50,'Convert\nComplex','horiz','left');
  Frame Status Conversion3 : Subsystem  mask(Frame Status Conversion){growRefPort=off, outframe=Sample-based}
      mask prompts: growRefPort "Inherit output frame status from Ref input port"; outframe "Output signal:"
      mask help: Specify the frame status of the output signal.
      mask init:
      | [p, str] = dspblkfrmconv('init');
      mask Help: web(dspbhelp);
      mask Callback growRefPort: dspblkfrmconv
      mask TypeOptions outframe: Frame-based | Sample-based
      mask Display:
      | port_label(p.in1,   p.i1,  p.i1s);
      | port_label(p.in2,   p.i2,  p.i2s);
      | port_label(p.out, p.o1, p.o1s);
      | disp(str)
  Frame Status Conversion4 : Subsystem  mask(Frame Status Conversion){growRefPort=off, outframe=Sample-based}
      mask prompts: growRefPort "Inherit output frame status from Ref input port"; outframe "Output signal:"
      mask help: Specify the frame status of the output signal.
      mask init:
      | [p, str] = dspblkfrmconv('init');
      mask Help: web(dspbhelp);
      mask Callback growRefPort: dspblkfrmconv
      mask TypeOptions outframe: Frame-based | Sample-based
      mask Display:
      | port_label(p.in1,   p.i1,  p.i1s);
      | port_label(p.in2,   p.i2,  p.i2s);
      | port_label(p.out, p.o1, p.o1s);
      | disp(str)
  Mux : Mux  Inputs=2
  S-Function simscopit : S-Function  FunctionName=sf1_simscopit2tr_Sept08  Parameters=name_plot,samplefreq,figpos,stemdo,upstartman,freqtickvec,1  EnableBusSupport=off
  Unbuffer : Unbuffer
  Unbuffer1 : Unbuffer
  wires:
  Frame Status Conversion4/1(Out) -> Convert Complex Simulink to DSP 1/1(In)
  Frame Status Conversion3/1(Out) -> "Convert Complex Simulink to DSP "/1(In)
  "Convert Complex Simulink to DSP "/1(Out) -> Mux/1
  Convert Complex Simulink to DSP 1/1(Out) -> Mux/2
  Unbuffer1/1 -> Buffer1/1
  Unbuffer/1 -> Buffer/1
  In2/1 -> Unbuffer1/1
  Mux/1 -> S-Function simscopit/1
  In1/1 -> Unbuffer/1
  Buffer1/1 -> Frame Status Conversion4/1(In1)
  Buffer/1 -> Frame Status Conversion3/1(In1)
